simulink model "DSPLab6"  (R2013a)
settings: Solver=ode45  StartTime=0.0  StopTime=10.0  RelTol=1e-3
undefined symbols (not defined in the file or in its folder): i
settings Model: Creator=M. Hassan  LastModifiedBy=M. Hassan

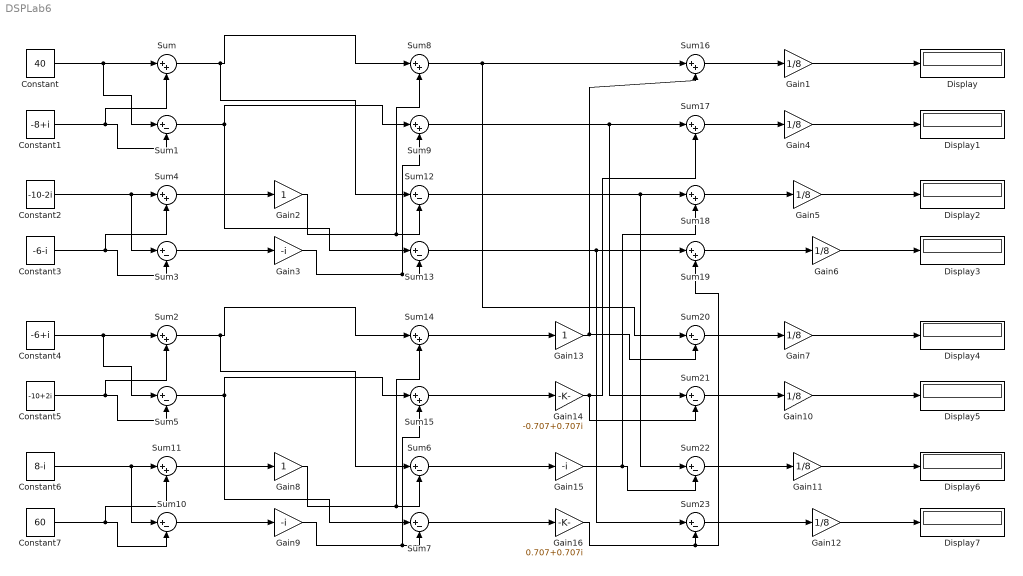
== system DSPLab6 ==
  Constant : Constant  Value=40
  Constant1 : Constant  Value=-8+i
  Constant2 : Constant  Value=-10-2i
  Constant3 : Constant  Value=-6-i
  Constant4 : Constant  Value=-6+i
  Constant5 : Constant  Value=-10+2i
  Constant6 : Constant  Value=8-i
  Constant7 : Constant  Value=60
  Display{,1..7} (8 alike) : Display
  Gain{1,4..7,10..12} (8 alike) : Gain  Gain=1/8
  Gain13 : Gain
  Gain14 : Gain  Gain=-0.707+0.707i
  Gain15 : Gain  Gain=-i
  Gain16 : Gain  Gain=0.707+0.707i
  Gain2 : Gain
  Gain3 : Gain  Gain=-i
  Gain8 : Gain
  Gain9 : Gain  Gain=-i
  Sum{,2,4,8..9,11,14..19} (12 alike) : Sum  Inputs=|++
  Sum{1,3,5..7,10,12..13,20..23} (12 alike) : Sum  Inputs=|+-
  wires:
  Constant/1 -> Sum1/1, Sum/1
  Constant1/1 -> Sum1/2, Sum/2
  Constant2/1 -> Sum3/1, Sum4/1
  Constant3/1 -> Sum3/2, Sum4/2
  Sum/1 -> Sum12/1, Sum8/1
  Sum1/1 -> Sum9/1, Sum13/1
  Sum4/1 -> Gain2/1
  Gain2/1 -> Sum8/2, Sum12/2
  Sum3/1 -> Gain3/1
  Gain3/1 -> Sum9/2, Sum13/2
  Gain1/1 -> Display/1
  Gain4/1 -> Display1/1
  Gain5/1 -> Display2/1
  Gain6/1 -> Display3/1
  Constant4/1 -> Sum5/1, Sum2/1
  Constant5/1 -> Sum5/2, Sum2/2
  Constant6/1 -> Sum10/1, Sum11/1
  Constant7/1 -> Sum10/2, Sum11/2
  Sum2/1 -> Sum6/1, Sum14/1
  Sum5/1 -> Sum15/1, Sum7/1
  Sum11/1 -> Gain8/1
  Gain8/1 -> Sum14/2, Sum6/2
  Sum10/1 -> Gain9/1
  Gain9/1 -> Sum15/2, Sum7/2
  Gain7/1 -> Display4/1
  Gain10/1 -> Display5/1
  Gain11/1 -> Display6/1
  Gain12/1 -> Display7/1
  Sum8/1 -> Sum20/1, Sum16/1
  Sum9/1 -> Sum17/1, Sum21/1
  Sum12/1 -> Sum22/1, Sum18/1
  Sum13/1 -> Sum19/1, Sum23/1
  Sum14/1 -> Gain13/1
  Gain13/1 -> Sum20/2, Sum16/2
  Sum15/1 -> Gain14/1
  Sum6/1 -> Gain15/1
  Gain15/1 -> Sum22/2, Sum18/2
  Sum7/1 -> Gain16/1
  Gain16/1 -> Sum23/2, Sum19/2
  Gain14/1 -> Sum17/2, Sum21/2
  Sum16/1 -> Gain1/1
  Sum17/1 -> Gain4/1
  Sum18/1 -> Gain5/1
  Sum19/1 -> Gain6/1
  Sum20/1 -> Gain7/1
  Sum21/1 -> Gain10/1
  Sum22/1 -> Gain11/1
  Sum23/1 -> Gain12/1
